simulink library "tether002_ul"  (R2020a)
settings: Solver=VariableStepAuto  StartTime=0.0  StopTime=10.0  RelTol=1e-3
values from neighbouring files (symbols this model uses):
  initNodePos = [INITIALLINE;INITIALLINE;INITIALLINE]    [tether002_ts.m]
  initNodeVel = [zeros(1,numNodes-2);zeros(1,numNodes-2);zeros(1,numNodes-2)]    [tether002_ts.m]
  numNodes = 11    [tether002_ts.m]
undefined symbols (not defined in the file or in its folder): TotoalNodes
libraries: powerlib_meascontrol x11, nodePosToLinkPos_ul x6, dspmtrx3 x4, sharedtransform x3, simulink_extras x2
(part 2 of 4)

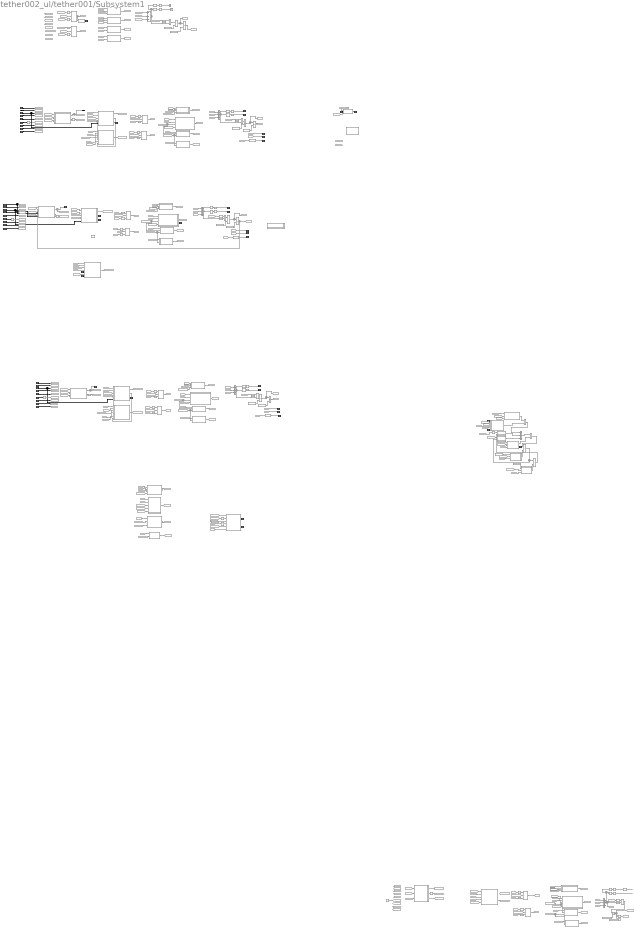
== system tether002_ul/tether001/Subsystem1 ==
  note: hysterisis first try
  note: Origional
  note: Current Edit
  note: "Dumbell" Edit
  In1 : Inport
  In2 : Inport  Port=2
  Veldata : Inport  Port=3
  airNodePos : Inport  Port=4
  In5 : Inport  Port=5
  In6 : Inport  Port=6
  In7 : Inport  Port=7
  In8 : Inport  Port=8
  In9 : Inport  Port=9
  In10 : Inport  Port=10
  gndNodePos : Inport  Port=11
  In12 : Inport  Port=12
  airNodePos1 : Inport  Port=13
  In14 : Inport  Port=14
  In15 : Inport  Port=15
  In16 : Inport  Port=16
  In17 : Inport  Port=17
  In18 : Inport  Port=18
  In19 : Inport  Port=19
  ActiveLengths : Inport  Port=20
  ReelInDirection : Inport  Port=21
  In22 : Inport  Port=22
  In23 : Inport  Port=23
  airNodePos2 : Inport  Port=24
  In25 : Inport  Port=25
  In26 : Inport  Port=26
  In27 : Inport  Port=27
  In28 : Inport  Port=28
  In29 : Inport  Port=29
  In30 : Inport  Port=30
  TotalForce : Inport  Port=31
  airNodePos3 : Inport  Port=32
  Add{,1..3,5..6} (6 alike) : Sum  Commented=on  Inputs=3
  Constant{1,3,5..6,8,10,13} (7 alike) : Constant  Commented=on  Value=initNodeVel
  Constant{2,4,7,9,14} (5 alike) : Constant  Commented=on  Value=initNodePos
  Constant17 : Constant  Commented=on  Value=[initNodeVel]
  Constant18 : Constant  Commented=on  Value=[initNodePos]
  Derivative : Derivative  Commented=on
  First-Order Filter : powerlib_meascontrol/Filters/First-Order Filter  Commented=on  FilterType=Lowpass  Tc=10e-3  Ts=.1  Initialize=on  Vac_Init=[0, 0, 60]  Vdc_Init=0  PlotResponse=off  FreqRange="[0,  200,  1]"
  First-Order Filter7 : powerlib_meascontrol/Filters/First-Order Filter  Commented=on  FilterType=Lowpass  Tc=.1  Ts=0  Initialize=on  Vac_Init=[0, 0, 60]  Vdc_Init=0  PlotResponse=off  FreqRange="[0,  200,  1]"
  From : From  Commented=on  GotoTag=CurrentLengths
  From{1,13,45,63,85,102,121,138,199,315,327} (11 alike) : From  Commented=on  GotoTag=gndNodePos
  From{3,9..10,114,150,335} (6 alike) : From  Commented=on  GotoTag=linkFlowVelVecs
  From{6,61,100,136,325} (5 alike) : From  Commented=on  GotoTag=FNetTen
  From{7,62,101,137,326} (5 alike) : From  Commented=on  GotoTag=FNetBuoy
  From{21,64,103,139,198,328} (6 alike) : From  Commented=on  GotoTag=midNodePos
  From{65,68,70..73,78,104,107,109..110,112,140,143,145..146,148,183,186,188,190,195,329,331..332,334} (26 alike) : From  Commented=on  GotoTag=ActiveNodes
  From{66,105,141,336} (4 alike) : From  Commented=on  GotoTag=midNodePosInternal
  From{23,39,46,67,76,86,106,122,142,316,337} (11 alike) : From  Commented=on  GotoTag=gndNodeVel
  From{54,69,75,77,94,108,111,130,144,147,193,330,333} (13 alike) : From  Commented=on  GotoTag=ActiveLengths
  From{4,11,14,17,20,26,29..30,41..42,49,55,57,81..82,89,95,97,117..118,125,131,133,312..313,322} (26 alike) : From  Commented=on  GotoTag=nodePos
  From{24,48,79,88,113,124,149,318} (8 alike) : From  Commented=on  GotoTag=airNodeVel
  From{2,59,115,175,185,187,189,194,310} (9 alike) : From  Commented=on  GotoTag=OriginalLengths
  From{35,80,116,311,338} (5 alike) : From  Commented=on  GotoTag=ReeledOutLength
  From{25,44,84,119..120,309} (6 alike) : From  Commented=on  GotoTag=midNodeVel
  From{5,12,15,27,50,56,58,74,90,96,98,126,132,134,321,323} (16 alike) : From  Commented=on  GotoTag=nodeVel
  From{19,47,87,123,317} (5 alike) : From  Commented=on  GotoTag=airNodePos
  From{8,37..38,51,91,127,184,319} (8 alike) : From  Commented=on  GotoTag=invNodeMasses
  From{16,22,40,52,92,128,320} (7 alike) : From  Commented=on  GotoTag=TetherLength
  From{53,93,129,191..192} (5 alike) : From  Commented=on  GotoTag=ReelInVel
  From{18,60,99,135,324} (5 alike) : From  Commented=on  GotoTag=FDrag
  From28 : From  Commented=on  GotoTag=CurrentLengths
  From31 : From  Commented=on  GotoTag=NumberNodesCurrent
  From314 : From  Commented=on  GotoTag=midNodeVelInternal
  From32 : From  Commented=on  GotoTag=NumberNodesActive
  From33 : From  Commented=on  GotoTag=NUMBEROFNODES
  From34 : From  Commented=on  GotoTag=CurrentLengths
  From36 : From  Commented=on  GotoTag=UnstrechedLengths
  From43 : From  Commented=on  GotoTag=midNodeVelInternal
  From83 : From  Commented=on  GotoTag=midNodeVelInternal
  Goto{,35,56,77,165} (5 alike) : Goto  Commented=on  GotoTag=gndNodePos
  Goto{1,26,46,67,157} (5 alike) : Goto  Commented=on  GotoTag=airNodePos
  Goto{10,33,54,75,145} (5 alike) : Goto  Commented=on  GotoTag=midNodeVel
  Goto{11,34,55,76,144} (5 alike) : Goto  Commented=on  GotoTag=midNodePos
  Goto{12,17,32,53,74,164} (6 alike) : Goto  Commented=on  GotoTag=FDrag
  Goto{13,18,31,52,73,163} (6 alike) : Goto  Commented=on  GotoTag=FNetTen
  Goto{14,19,30,51,72,162} (6 alike) : Goto  Commented=on  GotoTag=FNetBuoy
  Goto{8,37,58,79,146} (5 alike) : Goto  Commented=on  GotoTag=ReeledOutLength
  Goto{38,59,80,147} (4 alike) : Goto  Commented=on  GotoTag=OriginalLengths
  Goto{40,61,82,148} (4 alike) : Goto  Commented=on  GotoTag=ReelInVel
  Goto149 : Goto  Commented=on  GotoTag=Forces
  Goto{15,20,27,47,68,158} (6 alike) : Goto  Commented=on  GotoTag=invNodeMasses
  Goto150 : Goto  Commented=on  GotoTag=OriginalNodes
  Goto{39,60,81,151} (4 alike) : Goto  Commented=on  GotoTag=midNodeVelInternal
  Goto{21,41,62,152} (4 alike) : Goto  Commented=on  GotoTag=ActiveLengths
  Goto{6,22,42,63,153} (5 alike) : Goto  Commented=on  GotoTag=linkFlowVelVecs
  Goto{9,23,43,64,154} (5 alike) : Goto  Commented=on  GotoTag=nodePos
  Goto{5,24,44,65,155} (5 alike) : Goto  Commented=on  GotoTag=airNodeVel
  Goto{4,25,45,66,156} (5 alike) : Goto  Commented=on  GotoTag=gndNodeVel
  Goto{16,28,48,69,159} (5 alike) : Goto  Commented=on  GotoTag=nodeVel
  Goto{29,49,70,160} (4 alike) : Goto  Commented=on  GotoTag=TetherLength
  Goto{3,50,71,161} (4 alike) : Goto  Commented=on  GotoTag=ActiveNodes
  Goto{36,57,78,166} (4 alike) : Goto  Commented=on  GotoTag=midNodePosInternal
  Goto2 : Goto  Commented=on  GotoTag=TotalNodes
  Goto7 : Goto  Commented=on  GotoTag=unstretchedLength
  HowManyActive : MATLAB Function  Commented=on  TreatAsAtomicUnit=on
  HowManyActive1 : MATLAB Function  Commented=on  TreatAsAtomicUnit=on
  HowManyActive2 : MATLAB Function  Commented=on  TreatAsAtomicUnit=on
  HowManyActive4 : MATLAB Function  Commented=on  TreatAsAtomicUnit=on
  Hydrodynamic Force : Subsystem  Commented=on
  Hydrodynamic Force2 : Subsystem  Commented=on  AncestorBlock=tether002_ul/tether001/Hydrodynamic Force
  Integrator{,1..7,10..13} (12 alike) : Integrator  Commented=on  InitialConditionSource=external
  Inv Mass Matrix : Subsystem  Commented=on
  MATLAB Function : MATLAB Function  Commented=on  TreatAsAtomicUnit=on
  MATLAB Function1 : MATLAB Function  Commented=on  TreatAsAtomicUnit=on
  MATLAB Function10 : MATLAB Function  Commented=on  TreatAsAtomicUnit=on
  MATLAB Function11 : MATLAB Function  Commented=on  TreatAsAtomicUnit=on
  MATLAB Function12 : MATLAB Function  Commented=on  TreatAsAtomicUnit=on
  MATLAB Function13 : MATLAB Function  Commented=on  TreatAsAtomicUnit=on
  MATLAB Function14 : MATLAB Function  Commented=on  TreatAsAtomicUnit=on
  MATLAB Function15 : MATLAB Function  Commented=on  TreatAsAtomicUnit=on
  MATLAB Function16 : MATLAB Function  Commented=on  TreatAsAtomicUnit=on
  MATLAB Function17 : MATLAB Function  Commented=on  TreatAsAtomicUnit=on
  MATLAB Function18 : MATLAB Function  Commented=on  TreatAsAtomicUnit=on
  MATLAB Function19 : MATLAB Function  Commented=on  TreatAsAtomicUnit=on
  MATLAB Function2 : MATLAB Function  Commented=on  TreatAsAtomicUnit=on
  MATLAB Function20 : MATLAB Function  Commented=on  TreatAsAtomicUnit=on
  MATLAB Function21 : MATLAB Function  Commented=on  TreatAsAtomicUnit=on
  MATLAB Function22 : MATLAB Function  Commented=on  TreatAsAtomicUnit=on
  MATLAB Function28 : MATLAB Function  Commented=on  TreatAsAtomicUnit=on
  MATLAB Function29 : MATLAB Function  Commented=on  TreatAsAtomicUnit=on
  MATLAB Function3 : MATLAB Function  Commented=on  TreatAsAtomicUnit=on
  MATLAB Function30 : MATLAB Function  Commented=on  TreatAsAtomicUnit=on
  MATLAB Function31 : MATLAB Function  Commented=on  TreatAsAtomicUnit=on
  MATLAB Function32 : MATLAB Function  Commented=on  TreatAsAtomicUnit=on
  MATLAB Function33 : MATLAB Function  Commented=on  TreatAsAtomicUnit=on
  MATLAB Function35 : MATLAB Function  Commented=on  TreatAsAtomicUnit=on
  MATLAB Function4 : MATLAB Function  Commented=on  TreatAsAtomicUnit=on
  MATLAB Function5 : MATLAB Function  Commented=on  TreatAsAtomicUnit=on
  MATLAB Function54 : MATLAB Function  Commented=on  TreatAsAtomicUnit=on
  MATLAB Function55 : MATLAB Function  Commented=on  TreatAsAtomicUnit=on
  MATLAB Function56 : MATLAB Function  Commented=on  TreatAsAtomicUnit=on
  MATLAB Function57 : MATLAB Function  Commented=on  TreatAsAtomicUnit=on
  MATLAB Function58 : MATLAB Function  Commented=on  TreatAsAtomicUnit=on
  MATLAB Function6 : MATLAB Function  Commented=on  TreatAsAtomicUnit=on
  MATLAB Function7 : MATLAB Function  Commented=on  TreatAsAtomicUnit=on
  MATLAB Function8 : MATLAB Function  Commented=on  TreatAsAtomicUnit=on
  MATLAB Function9 : MATLAB Function  Commented=on  TreatAsAtomicUnit=on
  Matrix Concatenate{,1..7,14..15} (10 alike) : Concatenate  Commented=on  NumInputs=3  Mode=Multidimensional array  ConcatenateDimension=2
  Multiply{,1..3,5..7} (7 alike) : Product  Commented=on
  Reshape{1..12,15..18,21..26,29..30,33..34,41..44} (30 alike) : Reshape  Commented=on  OutputDimensionality=Column vector (2-D)
  Reshape{13..14,19..20,27..28,39..40} (8 alike) : Reshape  Commented=on  OutputDimensionality=Row vector (2-D)
  Selector{,1,8,12,23} (5 alike) : Selector  Commented=on  NumberOfDimensions=2  InputPortWidth=3  IndexOptions=Select all,Index vector (dialog)  Indices=[1 3],1  OutputSizes=1,1
  Selector{6..7,10..11,14..15,24..25} (8 alike) : Selector  Commented=on  NumberOfDimensions=2  InputPortWidth=3  IndexOptions=Select all,Index vector (dialog)  Indices=[1 3],2:numNodes-1  OutputSizes=1,1
  Selector{4..5,9,13,26} (5 alike) : Selector  Commented=on  NumberOfDimensions=2  InputPortWidth=3  IndexOptions=Select all,Starting index (dialog)  Indices=[1 3],numNodes  OutputSizes=1,1
  Selector2 : Selector  Commented=on  NumberOfDimensions=2  InputPortWidth=3  IndexOptions=Select all,Index vector (dialog)  Indices=[1 3],2:TotoalNodes-1  OutputSizes=1,1
  Selector3 : Selector  Commented=on  NumberOfDimensions=2  InputPortWidth=3  IndexOptions=Select all,Index vector (dialog)  Indices=[1 3],2:TotoalNodes-1  OutputSizes=1,1
  Tension : Subsystem  Commented=on
  Tension Reel In : MATLAB Function  Commented=on  TreatAsAtomicUnit=on
  Terminator : Terminator  Commented=on
  Terminator2 : Terminator  Commented=on
  Unit Delay : UnitDelay  Commented=on  SampleTime=-1  HasFrameUpgradeWarning=on
  Unit Delay1 : UnitDelay  Commented=on  SampleTime=-1  HasFrameUpgradeWarning=on
  Velocity Reset : MATLAB Function  Commented=on  TreatAsAtomicUnit=on
  Weigh/Boyancy : Subsystem  Commented=on
  nodePosToLinkPos{,1..3} (4 alike) : nodePosToLinkPos_ul/nodePosToLinkPos  Commented=on  SystemSampleTime=-1  Latency=0  AutoFrameSizeCalculation=off
  linkPositions : Outport
  ActiveNodes : Outport  Port=2
  node1NetFVec : Outport  Port=3
  midNodeVel : Outport  Port=4
  nodeNNetFVec : Outport  Port=5
  Na : Outport  Port=6
  nodePositions : Outport  Port=7
  nodeVelocities : Outport  Port=8
  linkPositions1 : Outport  Port=9
  ActiveNodes1 : Outport  Port=10
  node1NetFVec1 : Outport  Port=11
  nodeNNetFVec1 : Outport  Port=12
  ReelInDirection1 : Outport  Port=13
  Na1 : Outport  Port=14
  linkLength : Outport  Port=15
  nodePositions1 : Outport  Port=16
  nodeVelocities1 : Outport  Port=17
  linkPositions2 : Outport  Port=18
  node1NetFVec2 : Outport  Port=19
  ActiveNodes2 : Outport  Port=20
  nodeNNetFVec2 : Outport  Port=21
  Na2 : Outport  Port=22
  nodePositions2 : Outport  Port=23
  nodeVelocities2 : Outport  Port=24
  linkPositions3 : Outport  Port=25
  L : Outport  Port=26
  Out27 : Outport  Port=27
  Vo : Outport  Port=28
  wires:
  Constant10/1 -> Integrator7/2
  Selector15/1 -> Multiply3/1
  From63/1 -> MATLAB Function9/1(gndNodePos)
  MATLAB Function8/1(nodeForceVecs) -> Goto30/1
  From43/1 -> Matrix Concatenate1/2
  From55/1 -> nodePosToLinkPos/1
  From3/1 -> Hydrodynamic Force2/3(linkFlowVelVecs)
  From193/1 -> MATLAB Function35/1(ActiveLengths)
  From50/1 -> nodeVelocities/1  "nodeVelocities"
  Selector4/1 -> Reshape5/1
  Reshape4/1 -> Terminator/1
  From5/1 -> Hydrodynamic Force2/2(nodeVelocities)
  From58/1 -> MATLAB Function5/2(nodeVel)
  From65/1 -> MATLAB Function9/3(ActiveNodes)
  From22/1 -> Weigh/Boyancy/2(unstretchedLength)
  Selector9/1 -> Reshape18/1
  From184/1 -> MATLAB Function29/1(invNodeMasses)
  From105/1 -> Matrix Concatenate4/2
  From84/1 -> MATLAB Function1/2(midNodeVel)
  From96/1 -> MATLAB Function13/2(nodeVelocities)
  Constant2/1 -> Integrator1/2
  Hydrodynamic Force/1(nodeForceVecs) -> Goto12/1
  Tension Reel In/1(nodeForceVecs) -> Goto18/1
  From6/1 -> Add/2
  MATLAB Function7/1(nodeForceVecs) -> Goto32/1
  From16/1 -> Inv Mass Matrix/2(unstretchedLength)
  Add1/1 -> Selector5/1, Selector6/1, Selector1/1
  Selector7/1 -> Multiply1/1
  Integrator/1 -> Goto10/1, Integrator1/1
  Reshape11/1 -> node1NetFVec/1  "node1NetFVec"
  From38/1 -> MATLAB Function4/3(ZeroData)
  From13/1 -> Reshape6/1
  From15/1 -> Tension/2(nodeVelocities)
  From11/1 -> Hydrodynamic Force/1(nodePositions)
  From89/1 -> nodePositions2/1  "nodePositions"
  Hydrodynamic Force2/1(nodeForceVecs) -> Goto17/1
  TotalForce/1 -> MATLAB Function28/1(TotalForce)
  From198/1 -> MATLAB Function28/5(midNodePos)
  From142/1 -> MATLAB Function16/1(gndNodeVel)
  From52/1 -> HowManyActive/3(TetherLength)
  Selector/1 -> Reshape4/1
  From145/1 -> MATLAB Function17/4(NumberNodesActive)
  Selector11/1 -> Multiply2/1
  MATLAB Function30/1(Link1initNodeVel) -> Integrator10/2
  Reshape2/1 -> Matrix Concatenate/3
  Matrix Concatenate1/1 -> Goto28/1
  From98/1 -> MATLAB Function11/2(nodeVel)
  Integrator10/1 -> MATLAB Function33/2(Node01Vel), Integrator11/1
  From45/1 -> Reshape1/1
  Integrator2/1 -> Goto34/1
  Matrix Concatenate4/1 -> Goto43/1
  From31/1 -> MATLAB Function2/3(NumberNodesCurrent)
  MATLAB Function11/1(nodeForceVecs) -> Goto52/1
  From111/1 -> MATLAB Function12/1(Activelength)
  From24/1 -> Reshape9/1
  From40/1 -> Tension/3(unstretchedLength)
  From17/1 -> Weigh/Boyancy/1(nodePositions)
  In30/1 -> Goto61/1
  HowManyActive1/2(ActiveLengths) -> Reshape19/1
  Velocity Reset/2(Vo) -> Vo/1
  From61/1 -> Add1/2
  From/1 -> Tension Reel In/3(CurrentLengths)
  From20/1 -> Inv Mass Matrix/1(nodePositions)
  Reshape22/1 -> Matrix Concatenate5/1
  From110/1 -> MATLAB Function13/4(NumberNodesActive)
  From144/1 -> MATLAB Function17/3(ActiveLengths), MATLAB Function20/2(ActiveLengths)
  Selector3/1 -> Multiply/1
  From39/1 -> MATLAB Function4/1(gndNodeVel)
  From113/1 -> MATLAB Function1/4(airNodeVel)
  Reshape8/1 -> Matrix Concatenate3/1
  MATLAB Function28/1(Link1Forces) -> Multiply5/2
  Derivative/1 -> MATLAB Function32/1(ReelInAcc)
  From147/1 -> MATLAB Function18/1(Activelength)
  From51/1 -> Selector7/1
  HowManyActive2/1(ActiveNodes) -> ActiveNodes1/1, Goto71/1
  In28/1 -> Goto58/1
  MATLAB Function5/1(nodeForceVecs) -> Goto31/1
  From32/1 -> Tension Reel In/4(NumberNodesActive)
  Weigh/Boyancy/1(nodeForceVecs) -> Goto14/1
  From29/1 -> MATLAB Function2/1(nodePos)
  Integrator1/1 -> Goto11/1
  From27/1 -> Tension Reel In/2(nodeVel)
  From81/1 -> MATLAB Function13/1(nodePositions)
  MATLAB Function15/2(ReelInDirection) -> MATLAB Function1/7(ReelInDirection)
  Multiply7/1 -> Integrator10/1
  From30/1 -> MATLAB Function3/1(nodePos)
  From34/1 -> MATLAB Function2/2(CurrentLengths)
  From28/1 -> MATLAB Function3/2(Activelength)
  Selector6/1 -> Multiply1/2
  MATLAB Function6/1(invNodeMasses) -> Goto27/1
  From36/1 -> Tension Reel In/5(UnstrechedLengths)
  From23/1 -> Reshape8/1
  In5/1 -> Goto24/1
  From60/1 -> Add1/1
  From82/1 -> MATLAB Function14/1(nodePositions)
  Integrator11/1 -> MATLAB Function32/2(Node01Vel)
  Reshape6/1 -> Matrix Concatenate2/1
  airNodePos2/1 -> MATLAB Function15/5(airNodePos), Goto46/1
  Reshape14/1 -> Goto38/1
  MATLAB Function32/1(OUT2) -> Add5/2  "-ldd*x"
  From112/1 -> MATLAB Function12/2(ActiveNodes), MATLAB Function14/3(NumberNodesActive)
  In25/1 -> Goto44/1
  From62/1 -> Add1/3
  From47/1 -> Reshape2/1
  From88/1 -> Reshape16/1
  HowManyActive1/1(ActiveNodes) -> ActiveNodes2/1, Goto50/1
  Selector5/1 -> Reshape12/1
  From79/1 -> MATLAB Function10/4(airNodeVel)
  MATLAB Function4/1(midNodeVel) -> midNodeVel/1
  From33/1 -> Hydrodynamic Force2/4(NUMBEROFNODES)
  Tension/1("nodeForceVecs ") -> Goto13/1
  From8/1 -> Selector3/1
  From41/1 -> MATLAB Function7/1(nodePositions)
  From2/1 -> HowManyActive/1(OriginalLengths)
  From72/1 -> Velocity Reset/1(Current)
  From66/1 -> Matrix Concatenate/2
  From102/1 -> MATLAB Function15/1(gndNodePos)
  From64/1 -> MATLAB Function9/2(midNodePos)
  From57/1 -> MATLAB Function5/1(nodePos)
  From108/1 -> MATLAB Function11/3(ActiveLengths), MATLAB Function14/2(ActiveLengths)
  HowManyActive2/2(ActiveLengths) -> Reshape27/1
  From44/1 -> MATLAB Function10/2(midNodeVel)
  From74/1 -> Unit Delay1/1
  From12/1 -> Hydrodynamic Force/2(nodeVelocities)
  From73/1 -> Unit Delay/1
  Add/1 -> Selector2/1, Selector/1, Selector4/1
  From75/1 -> Velocity Reset/5(ActiveLengths)
  From76/1 -> Velocity Reset/6(gndNodeVel)
  Integrator3/1 -> Goto55/1
  MATLAB Function16/1(midNodeVelInternal) -> Goto81/1
  Unit Delay/1 -> Velocity Reset/2(Previous)
  From18/1 -> Add/1
  From149/1 -> MATLAB Function16/4(airNodeVel)
  Unit Delay1/1 -> Velocity Reset/4(nodeVel)
  From121/1 -> Reshape23/1
  Constant3/1 -> Velocity Reset/3(initNodeVel)
  From148/1 -> MATLAB Function18/2(ActiveNodes), MATLAB Function20/3(NumberNodesActive)
  From10/1 -> Hydrodynamic Force/3(linkFlowVelVecs)
  In7/1 -> Reshape14/1
  From68/1 -> MATLAB Function10/3(ActiveNodes)
  From114/1 -> MATLAB Function13/3(flowVel)
  MATLAB Function18/1(invNodeMasses) -> Goto68/1
  Selector13/1 -> Reshape26/1
  MATLAB Function9/1(midNodePosInternal) -> Goto36/1
  From69/1 -> MATLAB Function5/3(ActiveLengths), MATLAB Function8/2(ActiveLengths)
  Reshape13/1 -> Goto21/1
  From54/1 -> MATLAB Function9/4(ActiveLengths), MATLAB Function10/5(ActiveLengths)
  From14/1 -> Tension/1(nodePositions)
  Constant6/1 -> Integrator4/2
  From94/1 -> MATLAB Function15/4(ActiveLengths), MATLAB Function1/5(ActiveLengths)
  Inv Mass Matrix/1(invNodeMasses) -> Goto15/1
  In29/1 -> Goto49/1
  Add3/1 -> Selector13/1, Selector14/1, Selector12/1
  From7/1 -> Add/3
  MATLAB Function20/1(nodeForceVecs) -> Goto72/1
  From132/1 -> MATLAB Function19/2(nodeVelocities)
  From195/1 -> MATLAB Function35/3(ActiveNodes)
  From126/1 -> nodeVelocities1/1  "nodeVelocities"
  MATLAB Function3/1(invNodeMasses) -> Goto20/1
  From192/1 -> Derivative/1
  From143/1 -> MATLAB Function16/3(ActiveNodes)
  Reshape15/1 -> Matrix Concatenate4/1
  In10/1 -> Goto40/1
  MATLAB Function35/1(invL) -> Multiply7/2
  From191/1 -> MATLAB Function33/1(ReelInVel)
  airNodePos1/1 -> MATLAB Function21/5(airNodePos), HowManyActive2/6(airNodePos), Goto67/1
  In2/1 -> Goto25/1
  gndNodePos/1 -> HowManyActive2/4(gndNodePos), Goto77/1
  airNodePos/1 -> MATLAB Function9/5(airNodePos), Goto26/1
  ActiveLengths/1 -> MATLAB Function16/5(ActiveLengths)
  Reshape25/1 -> node1NetFVec1/1  "node1NetFVec"
  Matrix Concatenate6/1 -> Goto64/1
  Reshape23/1 -> Matrix Concatenate6/1
  Multiply3/1 -> Integrator7/1
  From25/1 -> Matrix Concatenate3/2
  Reshape30/1 -> Matrix Concatenate7/1
  From91/1 -> Selector11/1
  From95/1 -> nodePosToLinkPos2/1
  MATLAB Function31/1(Link1initNodePos) -> Integrator11/2
  From190/1 -> MATLAB Function31/3(ActiveNodes)
  From125/1 -> nodePositions1/1  "nodePositions"
  MATLAB Function13/1(nodeForceVecs) -> Goto53/1
  From118/1 -> MATLAB Function20/1(nodePositions)
  From49/1 -> nodePositions/1  "nodePositions"
  From185/1 -> MATLAB Function29/2(OriginalLengths)
  Selector12/1 -> Reshape25/1
  nodePosToLinkPos/1 -> linkPositions1/1  "linkPositions"
  Reshape21/1 -> Matrix Concatenate4/3
  From26/1 -> Tension Reel In/1(nodePos)
  Reshape5/1 -> Terminator2/1
  MATLAB Function17/2(linkLength) -> linkLength/1
  In9/1 -> Goto29/1
  From85/1 -> Reshape15/1
  From183/1 -> MATLAB Function28/3(ActiveNodes)
  MATLAB Function15/1(midNodePosInternal) -> Goto57/1
  From138/1 -> MATLAB Function21/1(gndNodePos)
  Integrator4/1 -> Goto33/1, Integrator2/1
  From93/1 -> MATLAB Function1/6(ReelInVel)
  From70/1 -> MATLAB Function5/4(NumberNodesActive)
  From186/1 -> MATLAB Function29/3(ActiveNodes)
  MATLAB Function33/1(OUT) -> Add5/3  "-2*ld*xd"
  From129/1 -> MATLAB Function16/6(ReelInVel)
  From107/1 -> MATLAB Function1/3(ActiveNodes)
  From53/1 -> MATLAB Function10/6(ReelInVel)
  HowManyActive/1(ActiveNodes) -> ActiveNodes/1, Goto3/1
  From101/1 -> Add2/3
  In26/1 -> Goto42/1
  From71/1 -> MATLAB Function7/4(NumberNodesActive)
  From21/1 -> Matrix Concatenate2/2
  MATLAB Function21/1(midNodePosInternal) -> Goto78/1
  nodePosToLinkPos3/1 -> linkPositions2/1  "linkPositions"
  HowManyActive/2(ActiveLengths) -> Reshape13/1
  Selector2/1 -> Multiply/2
  MATLAB Function9/2(ReelInDirection) -> MATLAB Function10/7(ReelInDirection)
  In16/1 -> Reshape28/1
  Multiply/1 -> Integrator/1
  MATLAB Function14/1(nodeForceVecs) -> Goto51/1
  From115/1 -> HowManyActive2/1(OriginalLengths)
  Reshape19/1 -> Goto41/1
  From120/1 -> MATLAB Function16/2(midNodeVel)
  Integrator6/1 -> HowManyActive2/5(midNodePos), Goto76/1
  From67/1 -> MATLAB Function10/1(gndNodeVel)
  Reshape20/1 -> Goto59/1
  From48/1 -> Reshape10/1
  From106/1 -> MATLAB Function1/1(gndNodeVel)
  From86/1 -> Reshape22/1
  Matrix Concatenate/1 -> Goto23/1
  Constant1/1 -> Integrator/2
  Selector8/1 -> Reshape17/1
  Reshape24/1 -> Matrix Concatenate7/3
  MATLAB Function19/1(nodeForceVecs) -> Goto74/1
  Matrix Concatenate2/1 -> nodePosToLinkPos1/1, Goto9/1
  Reshape12/1 -> nodeNNetFVec/1  "nodeNNetFVec"
  In27/1 -> Reshape20/1
  From87/1 -> Reshape21/1
  Add2/1 -> Selector9/1, Selector10/1, Selector8/1
  From109/1 -> MATLAB Function11/4(NumberNodesActive)
  In8/1 -> Goto37/1
  Selector10/1 -> Multiply2/2
  Constant14/1 -> MATLAB Function31/1(initNodePos)
  From133/1 -> MATLAB Function17/1(nodePos)
  From97/1 -> MATLAB Function11/1(nodePos)
  Constant7/1 -> Integrator3/2
  Reshape28/1 -> Goto80/1
  Velocity Reset/1(Out) -> Out27/1
  Matrix Concatenate7/1 -> Goto69/1
  In6/1 -> Goto22/1
  Reshape29/1 -> Matrix Concatenate6/3
  From92/1 -> HowManyActive1/3(TetherLength)
  From122/1 -> Reshape30/1
  Multiply1/1 -> Integrator4/1
  From99/1 -> Add2/1
  MATLAB Function29/1(Link1invNodeMasses) -> Multiply5/1
  From56/1 -> MATLAB Function7/2(nodeVelocities)
  MATLAB Function1/1(midNodeVelInternal) -> Goto60/1
  From100/1 -> Add2/2
  From9/1 -> MATLAB Function7/3(flowVel)
  From77/1 -> MATLAB Function6/1(Activelength)
  From128/1 -> HowManyActive2/3(TetherLength)
  From116/1 -> HowManyActive2/2(ReeledOutLength)
  Reshape27/1 -> Goto62/1
  airNodePos3/1 -> MATLAB Function28/6(airNodePos)
  From150/1 -> MATLAB Function19/3(flowVel)
  From123/1 -> Reshape29/1
  From136/1 -> Add3/2
  Constant4/1 -> Integrator2/2
  From59/1 -> HowManyActive1/1(OriginalLengths)
  From78/1 -> MATLAB Function6/2(ActiveNodes), MATLAB Function8/3(NumberNodesActive)
  MATLAB Function2/1(nodeForceVecs) -> Goto19/1
  From194/1 -> MATLAB Function35/2(OriginalLengths)
  From130/1 -> MATLAB Function21/4(ActiveLengths)
  Reshape9/1 -> Matrix Concatenate3/3
  MATLAB Function35/2(L) -> L/1
  From80/1 -> HowManyActive1/2(ReeledOutLength)
  Constant13/1 -> MATLAB Function30/1(initNodeVel)
  From139/1 -> MATLAB Function21/2(midNodePos)
  From188/1 -> MATLAB Function30/3(ActiveNodes)
  MATLAB Function17/1(nodeForceVecs) -> Goto73/1
  MATLAB Function10/1(midNodeVelInternal) -> Goto39/1
  In12/1 -> Goto66/1
  From124/1 -> Reshape24/1
  From83/1 -> Matrix Concatenate5/2
  From35/1 -> HowManyActive/2(ReeledOutLength)
  MATLAB Function21/3(Na) -> Na1/1
  From134/1 -> MATLAB Function17/2(nodeVel)
  Reshape26/1 -> nodeNNetFVec1/1  "nodeNNetFVec"
  From146/1 -> MATLAB Function19/4(NumberNodesActive)
  From140/1 -> MATLAB Function21/3(ActiveNodes)
  Constant9/1 -> Integrator6/2
  From131/1 -> nodePosToLinkPos3/1
  From46/1 -> Reshape3/1
  From137/1 -> Add3/3
  Integrator5/1 -> Goto54/1, Integrator3/1
  Reshape7/1 -> Matrix Concatenate2/3
  Reshape1/1 -> Matrix Concatenate/1
  Reshape10/1 -> Matrix Concatenate1/3
  From141/1 -> Matrix Concatenate6/2
  Reshape3/1 -> Matrix Concatenate1/1
  From135/1 -> Add3/1
  From119/1 -> Matrix Concatenate7/2
  From19/1 -> Reshape7/1
  From117/1 -> MATLAB Function19/1(nodePositions)
  From127/1 -> Selector15/1
  From199/1 -> MATLAB Function28/4(gndNodePos)
  Veldata/1 -> MATLAB Function4/2(Veldata)
  MATLAB Function12/1(invNodeMasses) -> Goto47/1
  Reshape17/1 -> node1NetFVec2/1  "node1NetFVec"
  Constant8/1 -> Integrator5/2
  From4/1 -> Hydrodynamic Force2/1(nodePositions)
  Integrator7/1 -> Goto75/1, Integrator6/1
  From42/1 -> MATLAB Function8/1(nodePositions)
  Reshape16/1 -> Matrix Concatenate5/3
  Reshape18/1 -> nodeNNetFVec2/1  "nodeNNetFVec"
  In14/1 -> Goto65/1
  From103/1 -> MATLAB Function15/2(midNodePos)
  Selector1/1 -> Reshape11/1
  Multiply5/1 -> Add5/1  "(1/m)*F"
  Selector14/1 -> Multiply3/2
  Multiply2/1 -> Integrator5/1
  Matrix Concatenate3/1 -> Goto16/1
  From104/1 -> MATLAB Function15/3(ActiveNodes)
  Matrix Concatenate5/1 -> Goto48/1
  Add5/1 -> Multiply7/1
  From187/1 -> MATLAB Function30/2(OriginalLengths)
  From175/1 -> MATLAB Function28/2(OriginalLengths)
  From189/1 -> MATLAB Function31/2(OriginalLengths)
  In15/1 -> Goto63/1
  In17/1 -> Goto79/1
  In18/1 -> Goto70/1
  From90/1 -> nodeVelocities2/1  "nodeVelocities"
  In19/1 -> Goto82/1
  In23/1 -> Goto45/1
  nodePosToLinkPos2/1 -> linkPositions3/1  "linkPositions"
  In22/1 -> Goto56/1
  MATLAB Function15/3(Na) -> Na2/1
  In1/1 -> Goto35/1
  nodePosToLinkPos1/1 -> linkPositions/1  "linkPositions"
  MATLAB Function9/3(Na) -> Na/1
  ReelInDirection/1 -> MATLAB Function16/7(ReelInDirection)
  MATLAB Function21/2(ReelInDirection) -> ReelInDirection1/1
  Integrator12/1 -> Goto145/1, Integrator13/1
  Constant17/1 -> Integrator12/2
  Constant18/1 -> Integrator13/2
  Integrator13/1 -> Goto144/1
  From309/1 -> MATLAB Function55/2(midNodeVel)
  MATLAB Function58/1(nodeForceVecs) -> Goto162/1
  From313/1 -> MATLAB Function58/1(nodePositions)
  From333/1 -> MATLAB Function56/1(Activelength)
  MATLAB Function57/1(nodeForceVecs) -> Goto164/1
  From335/1 -> MATLAB Function57/3(flowVel)
  From331/1 -> MATLAB Function54/5(NumberNodesActive)
  From322/1 -> MATLAB Function54/2(nodePos)
  From338/1 -> MATLAB Function54/1(ReeledOutLength)
  MATLAB Function55/2(midNodeVelInternal) -> Goto151/1
  From332/1 -> MATLAB Function57/4(NumberNodesActive)
  Multiply6/1 -> Integrator12/1
  MATLAB Function54/1(nodeForceVecs) -> Goto163/1
  From314/1 -> Matrix Concatenate14/2
  From318/1 -> Reshape34/1
  From321/1 -> MATLAB Function57/2(nodeVelocities)
  HowManyActive4/3(OriginalNodes) -> Goto150/1
  From320/1 -> HowManyActive4/3(TetherLength)
  From310/1 -> HowManyActive4/1(OriginalLengths)
  Reshape41/1 -> Matrix Concatenate15/3
  Reshape33/1 -> Matrix Concatenate15/1
  Reshape34/1 -> Matrix Concatenate14/3
  From328/1 -> MATLAB Function55/4(midNodePos)
  From327/1 -> MATLAB Function55/3(gndNodePos)
  From329/1 -> MATLAB Function55/5(ActiveNodes)
  From325/1 -> Add6/2
  From336/1 -> Matrix Concatenate15/2
  Selector25/1 -> Multiply6/1
  Selector24/1 -> Multiply6/2
  From311/1 -> HowManyActive4/2(ReeledOutLength)
  From330/1 -> MATLAB Function58/2(ActiveLengths), MATLAB Function54/4(ActiveLengths)
  Reshape42/1 -> Matrix Concatenate14/1
  Reshape40/1 -> Goto147/1
  Add6/1 -> Selector26/1, Selector23/1, Goto149/1, Selector24/1
  From324/1 -> Add6/1
  Matrix Concatenate15/1 -> Goto154/1
  HowManyActive4/1(ActiveNodes) -> Goto161/1
  Reshape43/1 -> First-Order Filter7/1  "node1NetFVec"
  Reshape44/1 -> ?  "nodeNNetFVec"
  Selector23/1 -> Reshape43/1
  Selector26/1 -> Reshape44/1
  From326/1 -> Add6/3
  First-Order Filter7/1 -> ?
  Matrix Concatenate14/1 -> Goto159/1
  Reshape39/1 -> Goto152/1
  From319/1 -> Selector25/1
  From334/1 -> MATLAB Function56/2(ActiveNodes), MATLAB Function58/3(NumberNodesActive)
  From323/1 -> MATLAB Function54/3(nodeVel)
  ? -> Goto157/1
  ? -> ?
  ? -> Goto156/1
  From317/1 -> Reshape41/1
  ? -> Goto165/1
  HowManyActive4/2(ActiveLengths) -> Reshape39/1
  From312/1 -> MATLAB Function57/1(nodePositions)
  ? -> Reshape40/1
  ? -> Goto146/1
  ? -> Goto155/1
  ? -> Goto160/1
  ? -> Goto153/1
  From337/1 -> MATLAB Function55/1(gndNodeVel)
  ? -> Goto148/1
  From315/1 -> Reshape33/1
  MATLAB Function56/1(invNodeMasses) -> Goto158/1
  From316/1 -> Reshape42/1

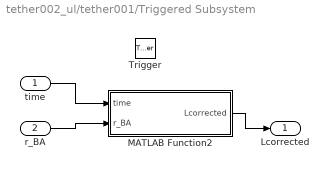
== system tether002_ul/tether001/Triggered Subsystem ==
  time : Inport
  r_BA : Inport  Port=2
  Trigger : TriggerPort  VariantControl=Variant
  MATLAB Function2 : MATLAB Function  TreatAsAtomicUnit=on
  Lcorrected : Outport
  wires:
  r_BA/1 -> MATLAB Function2/2(r_BA)
  time/1 -> MATLAB Function2/1(time)
  MATLAB Function2/1(Lcorrected) -> Lcorrected/1

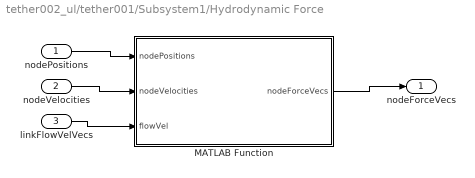
== system tether002_ul/tether001/Subsystem1/Hydrodynamic Force ==
  nodePositions : Inport
  nodeVelocities : Inport  Port=2
  linkFlowVelVecs : Inport  Port=3
  MATLAB Function : MATLAB Function  TreatAsAtomicUnit=on
  nodeForceVecs : Outport
  wires:
  nodePositions/1 -> MATLAB Function/1(nodePositions)
  linkFlowVelVecs/1 -> MATLAB Function/3(flowVel)
  MATLAB Function/1(nodeForceVecs) -> nodeForceVecs/1
  nodeVelocities/1 -> MATLAB Function/2(nodeVelocities)

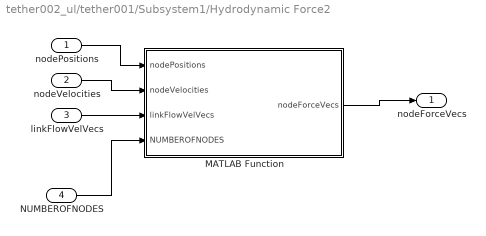
== system tether002_ul/tether001/Subsystem1/Hydrodynamic Force2 ==
  nodePositions : Inport
  nodeVelocities : Inport  Port=2
  linkFlowVelVecs : Inport  Port=3
  NUMBEROFNODES : Inport  Port=4
  MATLAB Function : MATLAB Function  TreatAsAtomicUnit=on
  nodeForceVecs : Outport
  wires:
  nodeVelocities/1 -> MATLAB Function/2(nodeVelocities)
  MATLAB Function/1(nodeForceVecs) -> nodeForceVecs/1
  linkFlowVelVecs/1 -> MATLAB Function/3(linkFlowVelVecs)
  nodePositions/1 -> MATLAB Function/1(nodePositions)
  NUMBEROFNODES/1 -> MATLAB Function/4(NUMBEROFNODES)

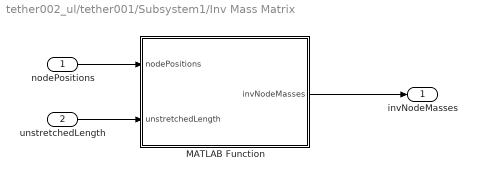
== system tether002_ul/tether001/Subsystem1/Inv Mass Matrix ==
  nodePositions : Inport
  unstretchedLength : Inport  Port=2
  MATLAB Function : MATLAB Function  TreatAsAtomicUnit=on
  invNodeMasses : Outport  VectorParamsAs1DForOutWhenUnconnected=off
  wires:
  nodePositions/1 -> MATLAB Function/1(nodePositions)
  unstretchedLength/1 -> MATLAB Function/2(unstretchedLength)
  MATLAB Function/1(invNodeMasses) -> invNodeMasses/1

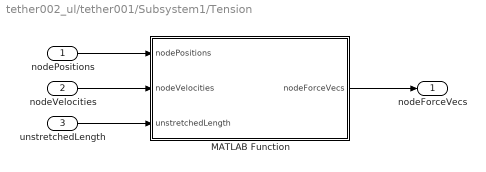
== system tether002_ul/tether001/Subsystem1/Tension ==
  nodePositions : Inport
  nodeVelocities : Inport  Port=2
  unstretchedLength : Inport  Port=3
  MATLAB Function : MATLAB Function  TreatAsAtomicUnit=on
  "nodeForceVecs " : Outport  VectorParamsAs1DForOutWhenUnconnected=off
  wires:
  nodeVelocities/1 -> MATLAB Function/2(nodeVelocities)
  unstretchedLength/1 -> MATLAB Function/3(unstretchedLength)
  nodePositions/1 -> MATLAB Function/1(nodePositions)
  MATLAB Function/1(nodeForceVecs) -> "nodeForceVecs "/1

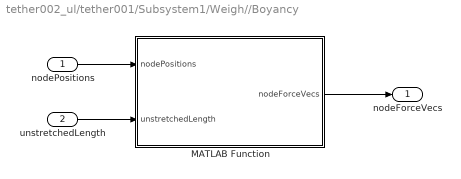
== system tether002_ul/tether001/Subsystem1/Weigh//Boyancy ==
  nodePositions : Inport
  unstretchedLength : Inport  Port=2
  MATLAB Function : MATLAB Function  TreatAsAtomicUnit=on
  nodeForceVecs : Outport  VectorParamsAs1DForOutWhenUnconnected=off
  wires:
  MATLAB Function/1(nodeForceVecs) -> nodeForceVecs/1
  unstretchedLength/1 -> MATLAB Function/2(unstretchedLength)
  nodePositions/1 -> MATLAB Function/1(nodePositions)

== matlab function tether002_ul/tether001/Subsystem1/MATLAB Function2 ==
  data: nodePos input; nodeForceVecs output; CurrentLengths input; NumberNodesCurrent input
function nodeForceVecs = fcn(nodePos, CurrentLengths,NumberNodesCurrent)

%clc
%clear
%CurrentLengths = [.5,1,2,2,4,2,1];

tetherDensity = 1300;
fluidDensity = 1000;
diameter = .0144;
gravity = 9.81;

nodeForceVecs  = zeros(1,11);

% In this notation, N is the number of nodes

% Length of each link 1xN-1
linkLengths = CurrentLengths(1:NumberNodesCurrent-1);

unstretchedLength = sum(linkLengths);

% Total length of all links, assuming they're straight lines, scalar
numericalTotalLength = sum(linkLengths);

% Number of links, scalar
numLinks = size(linkLengths,2);

% Total volume based on unspooled length, scalar
analyticalTotalVol  = unstretchedLength*(pi/4)*diameter^2;

% Total mass, based on unspooled length, scalar
analyticalTotalMass = tetherDensity*analyticalTotalVol;

% Mass of each link, 1xN-1
linkMasses  = analyticalTotalMass*(linkLengths./numericalTotalLength);

% Volume of each link, 1xN-1
linkVolumes = analyticalTotalVol*(linkLengths./numericalTotalLength);

% Net force on the links (buoyancy - gravity) on each link, 3xN-1
linkNetForceVecs = [repmat([0 0]',[1 numLinks]);(gravity*fluidDensity*linkVolumes-gravity*linkMasses)];

% Net force on the nodes, 3xN
nodeForceVecs = [linkNetForceVecs(:,1) linkNetForceVecs(:,1:end-1)+linkNetForceVecs(:,2:end) linkNetForceVecs(:,end)]/2;

== matlab function tether002_ul/tether001/Subsystem1/MATLAB Function3 ==
  data: nodePos input; invNodeMasses output; Activelength input
function invNodeMasses = fcn(nodePos,Activelength)
% 
% clc
% clear
% nodePos = [0,0,0,0,5,6.1,7.2,8.5,9.6,10,11;...
%            0,0,0,0,0,0  ,0  ,0  ,0  ,0 ,0 ;...
%            0,0,0,0,0,0  ,0  ,0  ,0  ,0 ,0 ];
% CurrentLengths = [0,0,0,1,1,1,1,1,1,1]';
% UnstrechedLengths = [1,1,1,1,1,1,1,1,1,1]';
% NumberNodesActive =10;
% TotalNodes = 11;

tetherDensity = 952;
diameter = .0144;

% In this notation, N is the number of nodes

unstretchedLength = sum(Activelength);

% Length of each link 1xN-1
linkLengths = sqrt(sum(diff(nodePos,1,2).^2));

% Total length of all links, assuming they're straight lines, scalar
numericalTotalLength = sum(linkLengths);

% Total volume based on current tether length, scalar
analyticalTotalVol  = unstretchedLength*(pi/4)*diameter^2;

% Total mass, based on current tether length, scalar
analyticalTotalMass = tetherDensity*analyticalTotalVol;

% Mass of each link, 1xN-1
linkMasses  = analyticalTotalMass*(linkLengths./numericalTotalLength);

% 1/mass for each node, 3xN (repmat so that we can multiply with force
% vectors concatenated into matrix later
invNodeMasses = repmat(1./([linkMasses(1) linkMasses(1:end-1)+linkMasses(2:end) linkMasses(end)]/2),[3 1]);

for i = 1:size(invNodeMasses,2)
    if invNodeMasses(:,i) == Inf
        invNodeMasses(:,i) = zeros(3,1);
    end
end

REALinvNodeMasses = zeros(size(invNodeMasses));
NonZeroRow = (find(invNodeMasses,1)+2)./3;

if NonZeroRow>1
    invNodeMasses(:,NonZeroRow)
    %REALinvNodeMasses(:,1) = invNodeMasses(:,NonZeroRow);
    %REALinvNodeMasses(:,NonZeroRow) = zeros(3,1);
end

invNodeMasses

== matlab function tether002_ul/tether001/Subsystem1/MATLAB Function ==
  data: gndNodePos input; midNodePos output; nodePos input; ZeroData input
function midNodePos = fcn(gndNodePos, nodePos, ZeroData)

% clc
% clear
% nodePos = [44,0,0,0,5,6.1,7.2,8.5,9.6,10,11;...
%            44,0,0,0,0,0  ,0  ,0  ,0  ,0 ,0 ;...
%            44,0,0,0,0,0  ,0  ,0  ,0  ,0 ,0 ];
% ZeroData = [1,0,0,0,1,1,1,1,1,1,1,1;...       
%             1,0,0,0,1,1,1,1,1,1,1,1;...  
%             1,0,0,0,1,1,1,1,1,1,1,1];
% gndNodePos = [99;99;99];        
% NumberNodesActive = 9;
% TotalNodes = 11;


correctedNodePos = zeros(size(nodePos));

for i = 1:size(nodePos,2)
    if ZeroData(:,i)==0
        correctedNodePos(:,i) = gndNodePos;
    else
        correctedNodePos(:,i) = nodePos(:,i);
    end
end

midNodePos = correctedNodePos;%(:,2:(end-1));

== matlab function tether002_ul/tether001/Subsystem1/MATLAB Function4 ==
  data: gndNodeVel input; midNodeVel output; Veldata input; ZeroData input
function midNodeVel = fcn(gndNodeVel, Veldata, ZeroData)

midNodeVel = zeros(size(Veldata));

for i = 1:size(Veldata,2)
    if ZeroData(:,i+1)==0
        midNodeVel(:,i) = gndNodeVel;
    else
        midNodeVel(:,i) = Veldata(:,i);
    end
end

midNodeVel = Veldata;

== matlab function tether002_ul/tether001/Subsystem1/MATLAB Function5 ==
  data: nodePos input; nodeForceVecs output; nodeVel input; ActiveLengths input; NumberNodesActive input
function nodeForceVecs = fcn(nodePos, nodeVel, ActiveLengths, NumberNodesActive)

% clc
% clear
% nodePos = [0,0,1,2,3,4,5,6,7,8,9;...
%            0,0,0,0,0,0,0,0,0,0,0;...
%            0,0,0,0,0,0,0,0,0,0,0];
% nodeVel = [1,1,1,1,0,0,0,0,0,0,0;...
%            1,1,1,1,0,0,0,0,0,0,0;...
%            1,1,1,1,0,0,0,0,0,0,0];       
% ActiveLengths = [0,0,.01,.1,.1,.1,.1,.1,.1,.1];
% NumberNodesActive = 9;
% TotalNodes = 11;

mass = .05;
zeta = .75;
diameter = .0144;
youngsMod = 5*10^10;

%Active = ActiveLengths(:,TotalNodes-NumberNodesActive+1);

TotalNodes = size(nodePos,2);

SpringConsts = [zeros(1,TotalNodes-NumberNodesActive+1),youngsMod*(pi/4)*(diameter^2)./ActiveLengths(1,(end-NumberNodesActive+3):end)];
%SpringConsts = [zeros(1,TotalNodes-NumberNodesActive+1),youngsMod*(pi/4)*(diameter^2)./ActiveLengths(1,(end-NumberNodesActive+3):end)];
DampCoeffs = zeta*2*sqrt(SpringConsts.*mass);

linkVecs  = diff(nodePos,1,2);

linkLength = sqrt(sum(linkVecs.^2));

linkUnitVecs = zeros(3,TotalNodes-1);
linkUnitVecs(1:3,(end-NumberNodesActive+2):end) = linkVecs(1:3,(end-NumberNodesActive+2):end)./repmat(sqrt(sum((linkVecs(1:3,(end-NumberNodesActive+2):end).^2),1)),[3 1]);

linkLengthDeriv = dot(nodeVel(:,2:end)-nodeVel(:,1:end-1),linkUnitVecs);

springForces = SpringConsts.*(linkLength-ActiveLengths);
damperForces = DampCoeffs.*linkLengthDeriv;

totalLinkForceVec = repmat(springForces+damperForces,[3 1]).*linkUnitVecs;

nodeForceVecs = [totalLinkForceVec(:,1) diff(totalLinkForceVec,1,2) -totalLinkForceVec(:,end)];

if SpringConsts(1) == 0
    nodeForceVecs(:,1) = nodeForceVecs(:,end-NumberNodesActive+2);
    nodeForceVecs(:,end-NumberNodesActive+2) = [0;0;0];
end

== matlab function tether002_ul/tether001/Subsystem1/MATLAB Function6 ==
  data: invNodeMasses output; Activelength input; ActiveNodes input
function invNodeMasses  = fcn(Activelength,ActiveNodes)
% clc
% clear
% Activelength = [0,0,.01,.1,.1,.1,.1,.1,.1,.1];
% ActiveNodes = 10;

tetherDensity = 952;
diameter = .0144;

% Mass of each link, 1xN-1
linkMasses  = tetherDensity*(Activelength*(pi/4)*diameter^2);

% 1/mass for each node, 3xN (repmat so that we can multiply with force
% vectors concatenated into matrix later
invNodeMasses = repmat(1./([linkMasses(1) linkMasses(1:end-1)+linkMasses(2:end) linkMasses(end)]/2),[3 1]);

%Make Zero Inverse mass also equal to zero
for i = 1:size(invNodeMasses,2)
    if invNodeMasses(:,i) == Inf
        invNodeMasses(:,i) = zeros(3,1);
    end
end

if invNodeMasses(:,1) == 0
    invNodeMasses(:,1) = invNodeMasses(:,end-ActiveNodes+2);
    invNodeMasses(:,end-ActiveNodes+2) = [0;0;0];
end




% REALinvNodeMasses = zeros(size(invNodeMasses));
% NonZeroRow = (find(invNodeMasses,1)+2)./3;

% if NonZeroRow>1
%     invNodeMasses(:,NonZeroRow);
%     %REALinvNodeMasses(:,1) = invNodeMasses(:,NonZeroRow);
%     %REALinvNodeMasses(:,NonZeroRow) = zeros(3,1);
% end






% tetherDensity = 952;
% diameter = .0144;
% 
% % Total Unstreched length of reeled out tether
% unstretchedLength = sum(Activelength);
% 
% % Length of each link based on active lengths 1xN-1
% linkLengths = Activelength;%linkLengths = sqrt(sum(diff(nodePos,1,2).^2));
% 
% % Total length of all links, assuming they're straight lines, scalar
% numericalTotalLength = sum(linkLengths);
% 
% % Total volume based on current tether length, scalar
% analyticalTotalVol  = unstretchedLength*(pi/4)*diameter^2;
% 
% % Total mass, based on current tether length, scalar
% analyticalTotalMass = tetherDensity*analyticalTotalVol;
% 
% % Mass of each link, 1xN-1
% linkMasses  = analyticalTotalMass*(linkLengths./numericalTotalLength);
% 
% % 1/mass for each node, 3xN (repmat so that we can multiply with force
% % vectors concatenated into matrix later
% invNodeMasses = repmat(1./([linkMasses(1) linkMasses(1:end-1)+linkMasses(2:end) linkMasses(end)]/2),[3 1]);
% 
% for i = 1:size(invNodeMasses,2)
%     if invNodeMasses(:,i) == Inf
%         invNodeMasses(:,i) = zeros(3,1);
%     end
% end
% 
% REALinvNodeMasses = zeros(size(invNodeMasses));
% NonZeroRow = (find(invNodeMasses,1)+2)./3;
% 
% if NonZeroRow>1
%     invNodeMasses(:,NonZeroRow);
%     %REALinvNodeMasses(:,1) = invNodeMasses(:,NonZeroRow);
%     %REALinvNodeMasses(:,NonZeroRow) = zeros(3,1);
% end
% 
% invNodeMasses
% end

== matlab function tether002_ul/tether001/Subsystem1/MATLAB Function7 ==
  data: nodePositions input; nodeForceVecs output; nodeVelocities input; flowVel input; NumberNodesActive input
function nodeForceVecs = fcn(nodePositions, nodeVelocities, flowVel,NumberNodesActive)
% In the notation here, N is the number of nodes, therefore you have N-1
% links between the nodes.

% N = 11;
% Length = 100;
% nodePositions = [zeros(1,N);linspace(1,Length,N);ones(1,N)];
% nodeVelocities = zeros(3,N);
% flowVel = [ones(1,N-1);.5*ones(1,N-1);.2*ones(1,N-1)];
% NumberNodesActive = 11;


flowDensity = 1025;
dragCoeff = .5;
thrDiam = .0144;

TotalNodes = size(nodePositions,2);

% Velocity and center of links 3xN-1
linkVelocities = (nodeVelocities(:,1:end-1) + nodeVelocities(:,2:end))/2;

% Apparent flow at center of links 3xN-1
linkAppFlow = flowVel - linkVelocities; %repmat(flowVel(:),[1 size(linkVelocities,2)]) - linkVelocities;
% linkAppFlow(3,:) = 0; % Origional model zeroed z component

% Link center apparent flow magnitude 3xN-1
linkAppFlowMag = sqrt(sum(linkAppFlow.^2)); % Sum over columns

% Normalize columns to get unit vector 3xN-1
dragDirUnitVec = linkAppFlow./repmat(linkAppFlowMag,[3 1]);
dragDirUnitVec(isnan(dragDirUnitVec)) = 0;

% If linkAppFlowMag is zero, dragDirUnitVec will have nans, patch to fix
% that with zeros
% dragDirUnitVec = zeros(3,numel(linkAppFlowMag==0));

% Dynamic pressures at link centers 1xN-1
dynPress = 0.5*flowDensity*linkAppFlowMag.^2;

linkVecs  = diff(nodePositions,1,2);

% Link lengths, diff over columns 1xN-1
linkLengths = sqrt(sum(diff(nodePositions,1,2).^2));

% Unit vectors in the direction of the link 3xN-1
linkUnitVecs = zeros(3,TotalNodes-1);
linkUnitVecs(1:3,(end-NumberNodesActive+2):end) = linkVecs(1:3,(end-NumberNodesActive+2):end)./repmat(sqrt(sum((linkVecs(1:3,(end-NumberNodesActive+2):end).^2),1)),[3 1]);

% Projected areas of each link
projArea = thrDiam*linkLengths.*sqrt(sum(cross(linkUnitVecs,dragDirUnitVec).^2,1));

% Drag force on links
linkForceVecs = repmat(dragCoeff*dynPress.*projArea,[3 1]).*dragDirUnitVec;

% Drag force on nodes
nodeForceVecs = [linkForceVecs(:,1) (linkForceVecs(:,1:end-1)+linkForceVecs(:,2:end)) linkForceVecs(:,end)]/2;

if NumberNodesActive<TotalNodes
    nodeForceVecs(:,1) = nodeForceVecs(:,end-NumberNodesActive+2);
    nodeForceVecs(:,end-NumberNodesActive+2) = [0;0;0];
end

== matlab function tether002_ul/tether001/Subsystem1/MATLAB Function8 ==
  data: nodePositions input; nodeForceVecs output; ActiveLengths input; NumberNodesActive input
function nodeForceVecs  = fcn(nodePositions, ActiveLengths, NumberNodesActive)

% clc
% clear
% nodePositions = [0,0,1,2,3,4,5,6,7,8,9;...
%            0,0,0,0,0,0,0,0,0,0,0;...
%            0,0,0,0,0,0,0,0,0,0,0];
%     
% ActiveLengths = [0,0,.01,.1,.1,.1,.1,.1,.1,.1];
% NumberNodesActive = 9;
% TotalNodes = 11;

tetherDensity = 952;
fluidDensity = 1025;
diameter = .0144;
gravity = 9.81;

% In this notation, N is the number of nodes

% Actual Length of each link 1xN-1
linkLengths = sqrt(sum(diff(nodePositions,1,2).^2));

% Number of links, scalar
numLinks = size(linkLengths,2);

% Volume of each link, 1xN-1
Volumes  = ActiveLengths.*(pi/4)*diameter^2;

% Mass of each link, 1xN-1
linkMasses = tetherDensity*Volumes;

% Net force on the links (buoyancy - gravity) on each link, 3xN-1
linkNetForceVecs = [repmat([0 0]',[1 numLinks]);(-gravity*linkMasses + gravity*fluidDensity*Volumes)];

% Net force on the nodes, 3xN
nodeForceVecs = [linkNetForceVecs(:,1) linkNetForceVecs(:,1:end-1)+linkNetForceVecs(:,2:end) linkNetForceVecs(:,end)]/2;

if linkMasses(1) == 0
    nodeForceVecs(:,1) = nodeForceVecs(:,end-NumberNodesActive+2);
    nodeForceVecs(:,end-NumberNodesActive+2) = [0;0;0];
end

== matlab function tether002_ul/tether001/Subsystem1/MATLAB Function9 ==
  data: gndNodePos input; midNodePosInternal output; midNodePos input; ActiveNodes input; ActiveLengths input; airNodePos input; ReelInDirection output; Na output
function [midNodePosInternal,ReelInDirection,Na] = fcn(gndNodePos, midNodePos, ActiveNodes, ActiveLengths, airNodePos)

% clc
% clear
% midNodePos = [1,2,3,4,5,6,7,8,9;...
%               1,2,3.5,4,5,6,7,8,9;...
%               1,2,3,4,5,6,7,8,9];
% ActiveLengths = [1.7,1.7,1.7,1.7,1.7,1.7,1.7,1.7,1.7];
% gndNodePos = [0;0;0];
% airNodePos = [10;10;10];
% ActiveNodes = 10;

%Radius = 15;

No = size(midNodePos,2)+2;
Na = ActiveNodes;

% if norm(midNodePos(:,(No-Na)+2))<Radius
%     Na = Na-1;
% end

% Reeled In Nodes are ground
midNodePosInternal = [gndNodePos(1)*ones(1,No-2);...
                      gndNodePos(2)*ones(1,No-2);...
                      gndNodePos(3)*ones(1,No-2)];

% Given for unalternd nodes
midNodePosInternal(:,((No-Na)+2):end) = midNodePos(:,((No-Na)+2):end);

% Find Vector between given nodes
midlinkVecs  = diff([midNodePosInternal,airNodePos],1,2);

% Find Unit Vector between given nodes
midlinkUnitVecs = midlinkVecs./repmat(sqrt(sum((midlinkVecs.^2),1)),[3 1]);

%Fixed length with slope of next link
%Option 1
midNodePosInternal(:,((No-Na)+1)) = gndNodePos+(ActiveLengths((No-Na)+1)*midlinkUnitVecs(:,(No-Na)+1));
ReelInDirection = midlinkUnitVecs(:,(No-Na)+1);

% Fixed length with slope of to top node
% Option 2
% a = diff([gndNodePos,airNodePos],1,2);
% MULT = a./repmat(sqrt(sum((a.^2),1)),[3 1]);
% midNodePosInternal(:,((No-Na)+1)) = gndNodePos+(ActiveLengths((No-Na)+1)*MULT);
% ReelInDirection = MULT;








% if No == Na
%     %All but first the same
%     midNodePosInternal(:,2:end) = midNodePos(:,2:end);
%     %length of first unstreched slope like the second
%     midNodePosInternal(:,1) = ActiveLengths(1)*midlinkUnitVecs(:,2);
% else

== matlab function tether002_ul/tether001/Subsystem1/MATLAB Function10 ==
  data: gndNodeVel input; midNodeVelInternal output; midNodeVel input; ActiveNodes input; airNodeVel input; ActiveLengths input; ReelInVel input; ReelInDirection input
function midNodeVelInternal = fcn(gndNodeVel,midNodeVel,ActiveNodes, airNodeVel, ActiveLengths, ReelInVel, ReelInDirection)

No = size(midNodeVel,2)+2;
Na = ActiveNodes;

midNodeVelInternal = [gndNodeVel(1)*ones(1,No-2);...
                      gndNodeVel(2)*ones(1,No-2);...
                      gndNodeVel(3)*ones(1,No-2)];

midNodeVelInternal(:,((No-Na)+2):end) = midNodeVel(:,((No-Na)+2):end);


nodeVelocities = [gndNodeVel,midNodeVel,airNodeVel];
linkVelocities = (nodeVelocities(:,1:end-1) + nodeVelocities(:,2:end))/2;


midNodeVelInternal(:,((No-Na)+1)) = -ReelInVel*ReelInDirection;


%midNodeVelInternal(:,((No-Na)+1)) = (linkVelocities(:,((No-Na)+1))*ActiveLengths(((No-Na)+1))+linkVelocities(:,((No-Na)+2))*ActiveLengths(((No-Na)+2)))/(ActiveLengths(((No-Na)+1))+ActiveLengths(((No-Na)+2)));




% if No == Na
%     midNodeVelInternal(:,:) = midNodeVel(:,(end-(ActiveNodes-3)):end);
% else
%     midNodeVelInternal(:,(end-(Na-3)):end) = midNodeVel(:,(end-(Na-3)):end);
% end

== matlab function tether002_ul/tether001/Subsystem1/Velocity Reset ==
  data: Current input; Out output; Previous input; initNodeVel input; Vo output; nodeVel input; ActiveLengths input; gndNodeVel input
function [Out,Vo] = fcn(Current, Previous, initNodeVel, nodeVel, ActiveLengths, gndNodeVel)

if Current == Previous
    Out = -1;
else
    Out = 1;
end
Vo = [gndNodeVel(1)*ones(1,length(ActiveLengths)-1);...
      gndNodeVel(2)*ones(1,length(ActiveLengths)-1);...
      gndNodeVel(3)*ones(1,length(ActiveLengths)-1)];

if all(ActiveLengths)
    Vo = initNodeVel;
else 
    Vo(1:3,(Previous-Current)+1:end-1) = nodeVel(1:3,2+(Previous-Current)+1:end-1);    
end
